simulink model "FlowInGasNetwork"  (R2023b)
settings: Solver=VariableStepAuto  StartTime=0.0  StopTime=10.0  RelTol=1e-3  AbsTol=1e-3
libraries: nesl_utility x6, fl_lib x5, simulink x4
(part 2 of 2)

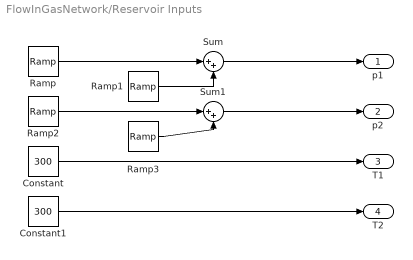
== system FlowInGasNetwork/Reservoir Inputs ==
  Constant : Constant  Value=300
  Constant1 : Constant  Value=300
  Ramp : simulink/Sources/Ramp  slope=0.1  start=6  InitialOutput=0.5
  Ramp1 : simulink/Sources/Ramp  slope=-0.1  start=9  InitialOutput=0
  Ramp2 : simulink/Sources/Ramp  slope=-0.075  start=1  InitialOutput=0.5
  Ramp3 : simulink/Sources/Ramp  slope=0.075  start=5  InitialOutput=0
  Sum : Sum  Inputs=|++
  Sum1 : Sum  Inputs=|++
  p1 : Outport
  p2 : Outport  Port=2
  T1 : Outport  Port=3
  T2 : Outport  Port=4
  wires:
  Constant/1 -> T1/1
  Constant1/1 -> T2/1
  Ramp1/1 -> Sum/2
  Ramp/1 -> Sum/1
  Sum/1 -> p1/1
  Sum1/1 -> p2/1
  Ramp2/1 -> Sum1/1
  Ramp3/1 -> Sum1/2

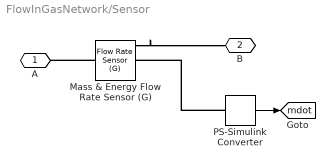
== system FlowInGasNetwork/Sensor ==
  Mass & Energy Flow Rate Sensor (G) : fl_lib/Gas/Sensors/Flow Rate Sensor (G)  mass_flow_measure=true  volumetric_flow_measure=false  volumetric_flow_conditions=foundation.enum.volumetric_flow_conditions.actual  p_std=0.101325 MPa  T_std=20 degC  energy_flow_measure=true
      settings: InternalSimscapePortConfiguration="{\"Bottom\":[{\"id\":\"PHI\",\"label\":\"φ\",\"type\":\"output\"}],\"Left\":[{\"id\":\"A\",\"label\":\"A\",\"type\":\"foundation.gas.gas\"}],\"Right\":[{\"id\":\"B\",\"label\":\"B\",\"type\":\"foundation.gas.gas\"},{\"id\":\"M\",\"label\":\"M\",\"type\":\"output\"}],\"Top\":[]}"
  PS-Simulink Converter : nesl_utility/PS-Simulink Converter  PhysicalDomain=network_engine_domain  SubClassName=ps_output  LeftPortType=input  RightPortType=output  PseudoPeriodic=off  Frequencies=[]  VectorFormat=1-D array  Unit=kg/s  AffineConversion=off
  A : PMIOPort  Side=Left
  B : PMIOPort  Port=2  Side=Right
  tag scope: mdot=global
  wires:
  PS-Simulink Converter/1 -> [mdot]
  connections:
  PS-Simulink Converter/LConn1 -- Mass & Energy Flow Rate Sensor (G)/RConn2
  Mass & Energy Flow Rate Sensor (G)/LConn1 -- A/RConn1
  Mass & Energy Flow Rate Sensor (G)/RConn1 -- B/RConn1
